simulink model "andmodel"  (R2023b)
settings: Solver=VariableStepAuto  StartTime=0.0  StopTime=10.0  RelTol=1e-3
settings Model: Creator=39216  LastModifiedBy=39216

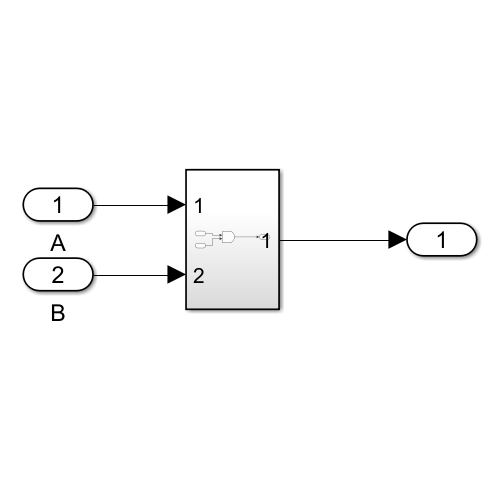
[thumbnail: Simulink's stored preview of the top-level diagram]
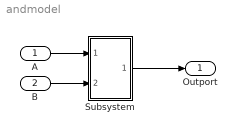
== system andmodel ==
  A : Inport
  B : Inport  Port=2
  Subsystem : Subsystem
  Outport : Outport
  wires:
  A/1 -> Subsystem/1(In1)
  B/1 -> Subsystem/2(In2)
  Subsystem/1(Out1) -> Outport/1

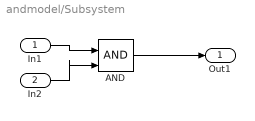
== system andmodel/Subsystem ==
  In1 : Inport
  In2 : Inport  Port=2
  AND : Logic  IconShape=distinctive  AllPortsSameDT=off  OutDataTypeStr=boolean
  Out1 : Outport
  wires:
  In1/1 -> AND/1
  AND/1 -> Out1/1
  In2/1 -> AND/2
